simulink model "lss"  (R2022b)
settings: Solver=FixedStepAuto  StartTime=0.0  StopTime=Inf  FixedStep=0.001  RelTol=1e-3  EnableMultiTasking=on
InitFcn:
  | clear mex
model workspace (MAT data in the model file):
  worldsim_instance : object (value not decoded)
values from neighbouring files (symbols this model uses):
  ADAS_Control_Mode = 1    [LSS_parameters.m]    (also in lss_ini_param.sldd = 1.0)
  butter_a = 1.0 -1.9911142922016536 0.99115359586893548    [lss_ini_param.sldd]
  butter_a_lka_out = 1.0 -1.5610180758007179 0.641351538057563    [lss_ini_param.sldd]
  butter_b = 9.825916820482009E-6 1.9651833640964018E-5 9.825916820482009E-6    [lss_ini_param.sldd]
  butter_b_lka_out = 0.020083365564211246 0.040166731128422492 0.020083365564211246    [lss_ini_param.sldd]
  index_variant_approaching_speed = 3.0    [lss_ini_param.sldd]
  initCond = vi_worldsim_load_scenario(worldsim_process,scenario_path,'lss_online')    [launcher.m]
  LDW_Activity_Flag = 1    [LSS_parameters.m]    (also in lss_ini_param.sldd = 1.0)
  LDW_Freq_Hz = Sensor_Freq_worldsim    [LSS_parameters.m]    (also in lss_ini_param.sldd = 50.0)
  LDW_LaneGap_dydt_Warning = 50    [LSS_parameters.m]    (also in lss_ini_param.sldd = 50.0)
  LDW_LaneGap_Warning = [0.5 0.25]    [LSS_parameters.m]    (also in lss_ini_param.sldd = 0.5 0.25)
  LDW_Min_Speed = 60    [LSS_parameters.m]    (also in lss_ini_param.sldd = 60.0)
  LDW_Steer_Vibration_Amplitude = 5    [LSS_parameters.m]    (also in lss_ini_param.sldd = 5.0)
  LDW_Steer_Vibration_Freq = 25    [LSS_parameters.m]    (also in lss_ini_param.sldd = 25.0)
  LKA_Activity_Flag = 1    [LSS_parameters.m]    (also in lss_ini_param.sldd = 1.0)
  LKA_D = [0.2 0.3]    [LSS_parameters.m]    (also in lss_ini_param.sldd = 0.2 0.3)
  LKA_Dyn_Rate_Limiter_Gain = 0.1    [LSS_parameters.m]    (also in lss_ini_param.sldd)
  LKA_Dyn_Rate_Limiter_Power = 10    [LSS_parameters.m]    (also in lss_ini_param.sldd = 10.0)
  LKA_Error_dydt_Off = 1    [LSS_parameters.m]    (also in lss_ini_param.sldd = 1.0)
  LKA_Error_Max = 3    [LSS_parameters.m]    (also in lss_ini_param.sldd = 3.0)
  LKA_Error_Off = 0.5    [LSS_parameters.m]    (also in lss_ini_param.sldd)
  LKA_Freq_Hz = Sensor_Freq_worldsim    [LSS_parameters.m]    (also in lss_ini_param.sldd = 50.0)
  LKA_I = [0.025 0.05]    [LSS_parameters.m]    (also in lss_ini_param.sldd = 0.025 0.05)
  LKA_Lane_Gap_Activate = [0.25 0.125]    [LSS_parameters.m]    (also in lss_ini_param.sldd = -0.05 0.125)
  LKA_Lane_Gap_dydt_Activate = 50    [LSS_parameters.m]    (also in lss_ini_param.sldd = 50.0)
  LKA_Min_Speed = 60    [LSS_parameters.m]    (also in lss_ini_param.mat = 50; lss_ini_param.sldd = 50.0)
  LKA_On_Display_Freq = 5    [LSS_parameters.m]    (also in lss_ini_param.sldd = 5.0)
  LKA_P = [0.1 0.2]    [LSS_parameters.m]    (also in lss_ini_param.sldd = 0.1 0.2)
  LKA_Steer_Rate_Max_radps = 1    [LSS_parameters.m]    (also in lss_ini_param.sldd = 1.0)
  radar_source = 2    [LSS_parameters.m]    (also in lss_ini_param.sldd = 2.0)
  Sensor_Freq_worldsim = 50    [launcher.m]    (also in lss_ini_param.sldd = 50.0)
  simulation_crt = '../VI-CarRealTime_model/SedanCar_WorldSim_Offline_send_svm.xml'    [launcher.m]
  stop_number_collisions = 5    [launcher.m]
  stop_speed = 0.001    [launcher.m]
  stop_time = 20    [launcher.m]
  target_speed = 72    [LSS_parameters.m]    (also in launcher.m = initCond.initialVelocity * 3.6)
  variant_approaching_speed = v_lat    [launcher.m]    (also in lss_ini_param.sldd = 0.2 0.3 0.4 0.5 0.6)
  vehicle_width = 1.86    [LSS_parameters.m]    (also in lss_ini_param.sldd = 2.05)
undefined symbols (not defined in the file or in its folder): Driver_Demands, light_brake_center, light_brake_left, light_brake_right, steer_assist, vicrt_initcallback, vicrt_initmexcallback, vicrt_simulationmanager
libraries: simulink x39, simwbSfunlib x15, viworldsim_lib x5
(part 6 of 6)

== system lss/VI-CarRealTime/Input_Bus/Inputs/Main_Spring/force ==
  BCforce : BusCreator  Inputs=4
  L1_def_val : Constant  Value=0
  L2_def_val : Constant  Value=0
  R1_def_val : Constant  Value=0
  R2_def_val : Constant  Value=0
  force : Outport
  wires:
  BCforce/1 -> force/1  "force"
  L1_def_val/1 -> BCforce/1  "L1"
  L2_def_val/1 -> BCforce/2  "L2"
  R1_def_val/1 -> BCforce/3  "R1"
  R2_def_val/1 -> BCforce/4  "R2"

== system lss/VI-CarRealTime/Input_Bus/Inputs/Mono_Element/Bumpstop_Damper ==
  BCBumpstop_Damper : BusCreator  Inputs=2
  front_def_val : Constant  Value=0
  rear_def_val : Constant  Value=0
  Bumpstop_Damper : Outport
  wires:
  BCBumpstop_Damper/1 -> Bumpstop_Damper/1  "Bumpstop_Damper"
  front_def_val/1 -> BCBumpstop_Damper/1  "front"
  rear_def_val/1 -> BCBumpstop_Damper/2  "rear"

== system lss/VI-CarRealTime/Input_Bus/Inputs/Mono_Element/Bumpstop_Damper_activity_flag ==
  BCBumpstop_Damper_activity_flag : BusCreator  Inputs=2
  front_def_val : Constant
  rear_def_val : Constant
  Bumpstop_Damper_activity_flag : Outport
  wires:
  BCBumpstop_Damper_activity_flag/1 -> Bumpstop_Damper_activity_flag/1  "Bumpstop_Damper_activity_flag"
  front_def_val/1 -> BCBumpstop_Damper_activity_flag/1  "front"
  rear_def_val/1 -> BCBumpstop_Damper_activity_flag/2  "rear"

== system lss/VI-CarRealTime/Input_Bus/Inputs/Mono_Element/Bumpstop_Spring ==
  BCBumpstop_Spring : BusCreator  Inputs=2
  front_def_val : Constant  Value=0
  rear_def_val : Constant  Value=0
  Bumpstop_Spring : Outport
  wires:
  BCBumpstop_Spring/1 -> Bumpstop_Spring/1  "Bumpstop_Spring"
  front_def_val/1 -> BCBumpstop_Spring/1  "front"
  rear_def_val/1 -> BCBumpstop_Spring/2  "rear"

== system lss/VI-CarRealTime/Input_Bus/Inputs/Mono_Element/Bumpstop_Spring_activity_flag ==
  BCBumpstop_Spring_activity_flag : BusCreator  Inputs=2
  front_def_val : Constant
  rear_def_val : Constant
  Bumpstop_Spring_activity_flag : Outport
  wires:
  BCBumpstop_Spring_activity_flag/1 -> Bumpstop_Spring_activity_flag/1  "Bumpstop_Spring_activity_flag"
  front_def_val/1 -> BCBumpstop_Spring_activity_flag/1  "front"
  rear_def_val/1 -> BCBumpstop_Spring_activity_flag/2  "rear"

== system lss/VI-CarRealTime/Input_Bus/Inputs/Mono_Element/Damper ==
  BCDamper : BusCreator  Inputs=2
  front_def_val : Constant  Value=0
  rear_def_val : Constant  Value=0
  Damper : Outport
  wires:
  BCDamper/1 -> Damper/1  "Damper"
  front_def_val/1 -> BCDamper/1  "front"
  rear_def_val/1 -> BCDamper/2  "rear"

== system lss/VI-CarRealTime/Input_Bus/Inputs/Mono_Element/Damper_activity_flag ==
  BCDamper_activity_flag : BusCreator  Inputs=2
  front_def_val : Constant
  rear_def_val : Constant
  Damper_activity_flag : Outport
  wires:
  BCDamper_activity_flag/1 -> Damper_activity_flag/1  "Damper_activity_flag"
  front_def_val/1 -> BCDamper_activity_flag/1  "front"
  rear_def_val/1 -> BCDamper_activity_flag/2  "rear"

== system lss/VI-CarRealTime/Input_Bus/Inputs/Mono_Element/Inerter ==
  BCInerter : BusCreator  Inputs=2
  front_def_val : Constant  Value=0
  rear_def_val : Constant  Value=0
  Inerter : Outport
  wires:
  BCInerter/1 -> Inerter/1  "Inerter"
  front_def_val/1 -> BCInerter/1  "front"
  rear_def_val/1 -> BCInerter/2  "rear"

== system lss/VI-CarRealTime/Input_Bus/Inputs/Mono_Element/Inerter_activity_flag ==
  BCInerter_activity_flag : BusCreator  Inputs=2
  front_def_val : Constant
  rear_def_val : Constant
  Inerter_activity_flag : Outport
  wires:
  BCInerter_activity_flag/1 -> Inerter_activity_flag/1  "Inerter_activity_flag"
  front_def_val/1 -> BCInerter_activity_flag/1  "front"
  rear_def_val/1 -> BCInerter_activity_flag/2  "rear"

== system lss/VI-CarRealTime/Input_Bus/Inputs/Mono_Element/Reboundstop_Damper ==
  BCReboundstop_Damper : BusCreator  Inputs=2
  front_def_val : Constant  Value=0
  rear_def_val : Constant  Value=0
  Reboundstop_Damper : Outport
  wires:
  BCReboundstop_Damper/1 -> Reboundstop_Damper/1  "Reboundstop_Damper"
  front_def_val/1 -> BCReboundstop_Damper/1  "front"
  rear_def_val/1 -> BCReboundstop_Damper/2  "rear"

== system lss/VI-CarRealTime/Input_Bus/Inputs/Mono_Element/Reboundstop_Damper_activity_flag ==
  BCReboundstop_Damper_activity_flag : BusCreator  Inputs=2
  front_def_val : Constant
  rear_def_val : Constant
  Reboundstop_Damper_activity_flag : Outport
  wires:
  BCReboundstop_Damper_activity_flag/1 -> Reboundstop_Damper_activity_flag/1  "Reboundstop_Damper_activity_flag"
  front_def_val/1 -> BCReboundstop_Damper_activity_flag/1  "front"
  rear_def_val/1 -> BCReboundstop_Damper_activity_flag/2  "rear"

== system lss/VI-CarRealTime/Input_Bus/Inputs/Mono_Element/Reboundstop_Spring ==
  BCReboundstop_Spring : BusCreator  Inputs=2
  front_def_val : Constant  Value=0
  rear_def_val : Constant  Value=0
  Reboundstop_Spring : Outport
  wires:
  BCReboundstop_Spring/1 -> Reboundstop_Spring/1  "Reboundstop_Spring"
  front_def_val/1 -> BCReboundstop_Spring/1  "front"
  rear_def_val/1 -> BCReboundstop_Spring/2  "rear"

== system lss/VI-CarRealTime/Input_Bus/Inputs/Mono_Element/Reboundstop_Spring_activity_flag ==
  BCReboundstop_Spring_activity_flag : BusCreator  Inputs=2
  front_def_val : Constant
  rear_def_val : Constant
  Reboundstop_Spring_activity_flag : Outport
  wires:
  BCReboundstop_Spring_activity_flag/1 -> Reboundstop_Spring_activity_flag/1  "Reboundstop_Spring_activity_flag"
  front_def_val/1 -> BCReboundstop_Spring_activity_flag/1  "front"
  rear_def_val/1 -> BCReboundstop_Spring_activity_flag/2  "rear"

== system lss/VI-CarRealTime/Input_Bus/Inputs/Mono_Element/Roll_Damper ==
  BCRoll_Damper : BusCreator  Inputs=2
  front_def_val : Constant  Value=0
  rear_def_val : Constant  Value=0
  Roll_Damper : Outport
  wires:
  BCRoll_Damper/1 -> Roll_Damper/1  "Roll_Damper"
  front_def_val/1 -> BCRoll_Damper/1  "front"
  rear_def_val/1 -> BCRoll_Damper/2  "rear"

== system lss/VI-CarRealTime/Input_Bus/Inputs/Mono_Element/Roll_Damper_activity_flag ==
  BCRoll_Damper_activity_flag : BusCreator  Inputs=2
  front_def_val : Constant
  rear_def_val : Constant
  Roll_Damper_activity_flag : Outport
  wires:
  BCRoll_Damper_activity_flag/1 -> Roll_Damper_activity_flag/1  "Roll_Damper_activity_flag"
  front_def_val/1 -> BCRoll_Damper_activity_flag/1  "front"
  rear_def_val/1 -> BCRoll_Damper_activity_flag/2  "rear"

== system lss/VI-CarRealTime/Input_Bus/Inputs/Mono_Element/Spring ==
  BCSpring : BusCreator  Inputs=2
  front_def_val : Constant  Value=0
  rear_def_val : Constant  Value=0
  Spring : Outport
  wires:
  BCSpring/1 -> Spring/1  "Spring"
  front_def_val/1 -> BCSpring/1  "front"
  rear_def_val/1 -> BCSpring/2  "rear"

== system lss/VI-CarRealTime/Input_Bus/Inputs/Mono_Element/Spring_activity_flag ==
  BCSpring_activity_flag : BusCreator  Inputs=2
  front_def_val : Constant
  rear_def_val : Constant
  Spring_activity_flag : Outport
  wires:
  BCSpring_activity_flag/1 -> Spring_activity_flag/1  "Spring_activity_flag"
  front_def_val/1 -> BCSpring_activity_flag/1  "front"
  rear_def_val/1 -> BCSpring_activity_flag/2  "rear"

== system lss/VI-CarRealTime/Input_Bus/Inputs/Rear_Steering_Actuator_disp/str_swa ==
  BCstr_swa : BusCreator  Inputs=2
  left_def_val : Constant  Value=0
  right_def_val : Constant  Value=0
  str_swa : Outport
  wires:
  BCstr_swa/1 -> str_swa/1  "str_swa"
  left_def_val/1 -> BCstr_swa/1  "left"
  right_def_val/1 -> BCstr_swa/2  "right"

== system lss/VI-CarRealTime/Input_Bus/Inputs/Steering/steer_at_spindle ==
  BCsteer_at_spindle : BusCreator  Inputs=4
  L1_def_val : Constant  Value=0
  L2_def_val : Constant  Value=0
  R1_def_val : Constant  Value=0
  R2_def_val : Constant  Value=0
  steer_at_spindle : Outport
  wires:
  BCsteer_at_spindle/1 -> steer_at_spindle/1  "steer_at_spindle"
  L1_def_val/1 -> BCsteer_at_spindle/1  "L1"
  L2_def_val/1 -> BCsteer_at_spindle/2  "L2"
  R1_def_val/1 -> BCsteer_at_spindle/3  "R1"
  R2_def_val/1 -> BCsteer_at_spindle/4  "R2"

== system lss/VI-CarRealTime/Input_Bus/Inputs/Subsystem_Activation/Internal_Brake_System_Activity ==
  BCInternal_Brake_System_Activity : BusCreator  Inputs=4
  L1_def_val : Constant
  L2_def_val : Constant
  R1_def_val : Constant
  R2_def_val : Constant
  Internal_Brake_System_Activity : Outport
  wires:
  BCInternal_Brake_System_Activity/1 -> Internal_Brake_System_Activity/1  "Internal_Brake_System_Activity"
  L1_def_val/1 -> BCInternal_Brake_System_Activity/1  "L1"
  L2_def_val/1 -> BCInternal_Brake_System_Activity/2  "L2"
  R1_def_val/1 -> BCInternal_Brake_System_Activity/3  "R1"
  R2_def_val/1 -> BCInternal_Brake_System_Activity/4  "R2"

== system lss/VI-CarRealTime/Input_Bus/Inputs/Subsystem_Activation/Tire_Force_x ==
  BCTire_Force_x : BusCreator  Inputs=4
  L1_def_val : Constant
  L2_def_val : Constant
  R1_def_val : Constant
  R2_def_val : Constant
  Tire_Force_x : Outport
  wires:
  BCTire_Force_x/1 -> Tire_Force_x/1  "Tire_Force_x"
  L1_def_val/1 -> BCTire_Force_x/1  "L1"
  L2_def_val/1 -> BCTire_Force_x/2  "L2"
  R1_def_val/1 -> BCTire_Force_x/3  "R1"
  R2_def_val/1 -> BCTire_Force_x/4  "R2"

== system lss/VI-CarRealTime/Input_Bus/Inputs/Subsystem_Activation/Tire_Force_y ==
  BCTire_Force_y : BusCreator  Inputs=4
  L1_def_val : Constant
  L2_def_val : Constant
  R1_def_val : Constant
  R2_def_val : Constant
  Tire_Force_y : Outport
  wires:
  BCTire_Force_y/1 -> Tire_Force_y/1  "Tire_Force_y"
  L1_def_val/1 -> BCTire_Force_y/1  "L1"
  L2_def_val/1 -> BCTire_Force_y/2  "L2"
  R1_def_val/1 -> BCTire_Force_y/3  "R1"
  R2_def_val/1 -> BCTire_Force_y/4  "R2"

== system lss/VI-CarRealTime/Input_Bus/Inputs/Subsystem_Activation/Tire_Force_z ==
  BCTire_Force_z : BusCreator  Inputs=4
  L1_def_val : Constant
  L2_def_val : Constant
  R1_def_val : Constant
  R2_def_val : Constant
  Tire_Force_z : Outport
  wires:
  BCTire_Force_z/1 -> Tire_Force_z/1  "Tire_Force_z"
  L1_def_val/1 -> BCTire_Force_z/1  "L1"
  L2_def_val/1 -> BCTire_Force_z/2  "L2"
  R1_def_val/1 -> BCTire_Force_z/3  "R1"
  R2_def_val/1 -> BCTire_Force_z/4  "R2"

== system lss/VI-CarRealTime/Input_Bus/Inputs/Subsystem_Activation/Tire_Moment_x ==
  BCTire_Moment_x : BusCreator  Inputs=4
  L1_def_val : Constant
  L2_def_val : Constant
  R1_def_val : Constant
  R2_def_val : Constant
  Tire_Moment_x : Outport
  wires:
  BCTire_Moment_x/1 -> Tire_Moment_x/1  "Tire_Moment_x"
  L1_def_val/1 -> BCTire_Moment_x/1  "L1"
  L2_def_val/1 -> BCTire_Moment_x/2  "L2"
  R1_def_val/1 -> BCTire_Moment_x/3  "R1"
  R2_def_val/1 -> BCTire_Moment_x/4  "R2"

== system lss/VI-CarRealTime/Input_Bus/Inputs/Subsystem_Activation/Tire_Moment_y ==
  BCTire_Moment_y : BusCreator  Inputs=4
  L1_def_val : Constant
  L2_def_val : Constant
  R1_def_val : Constant
  R2_def_val : Constant
  Tire_Moment_y : Outport
  wires:
  BCTire_Moment_y/1 -> Tire_Moment_y/1  "Tire_Moment_y"
  L1_def_val/1 -> BCTire_Moment_y/1  "L1"
  L2_def_val/1 -> BCTire_Moment_y/2  "L2"
  R1_def_val/1 -> BCTire_Moment_y/3  "R1"
  R2_def_val/1 -> BCTire_Moment_y/4  "R2"

== system lss/VI-CarRealTime/Input_Bus/Inputs/Subsystem_Activation/Tire_Moment_z ==
  BCTire_Moment_z : BusCreator  Inputs=4
  L1_def_val : Constant
  L2_def_val : Constant
  R1_def_val : Constant
  R2_def_val : Constant
  Tire_Moment_z : Outport
  wires:
  BCTire_Moment_z/1 -> Tire_Moment_z/1  "Tire_Moment_z"
  L1_def_val/1 -> BCTire_Moment_z/1  "L1"
  L2_def_val/1 -> BCTire_Moment_z/2  "L2"
  R1_def_val/1 -> BCTire_Moment_z/3  "R1"
  R2_def_val/1 -> BCTire_Moment_z/4  "R2"

== system lss/VI-CarRealTime/Input_Bus/Inputs/Third_Element/Damper_activity_flag ==
  BCDamper_activity_flag : BusCreator  Inputs=2
  front_def_val : Constant
  rear_def_val : Constant
  Damper_activity_flag : Outport
  wires:
  BCDamper_activity_flag/1 -> Damper_activity_flag/1  "Damper_activity_flag"
  front_def_val/1 -> BCDamper_activity_flag/1  "front"
  rear_def_val/1 -> BCDamper_activity_flag/2  "rear"

== system lss/VI-CarRealTime/Input_Bus/Inputs/Third_Element/Damper_force ==
  BCDamper_force : BusCreator  Inputs=2
  front_def_val : Constant  Value=0
  rear_def_val : Constant  Value=0
  Damper_force : Outport
  wires:
  BCDamper_force/1 -> Damper_force/1  "Damper_force"
  front_def_val/1 -> BCDamper_force/1  "front"
  rear_def_val/1 -> BCDamper_force/2  "rear"

== system lss/VI-CarRealTime/Input_Bus/Inputs/Third_Element/Spring ==
  BCSpring : BusCreator  Inputs=2
  front_def_val : Constant  Value=0
  rear_def_val : Constant  Value=0
  Spring : Outport
  wires:
  BCSpring/1 -> Spring/1  "Spring"
  front_def_val/1 -> BCSpring/1  "front"
  rear_def_val/1 -> BCSpring/2  "rear"

== system lss/VI-CarRealTime/Input_Bus/Inputs/Third_Element/Spring_activity_flag ==
  BCSpring_activity_flag : BusCreator  Inputs=2
  front_def_val : Constant
  rear_def_val : Constant
  Spring_activity_flag : Outport
  wires:
  BCSpring_activity_flag/1 -> Spring_activity_flag/1  "Spring_activity_flag"
  front_def_val/1 -> BCSpring_activity_flag/1  "front"
  rear_def_val/1 -> BCSpring_activity_flag/2  "rear"

== system lss/VI-CarRealTime/Input_Bus/Inputs/Tire_Force/Fx ==
  BCFx : BusCreator  Inputs=4
  L1_def_val : Constant  Value=0
  L2_def_val : Constant  Value=0
  R1_def_val : Constant  Value=0
  R2_def_val : Constant  Value=0
  Fx : Outport
  wires:
  BCFx/1 -> Fx/1  "Fx"
  L1_def_val/1 -> BCFx/1  "L1"
  L2_def_val/1 -> BCFx/2  "L2"
  R1_def_val/1 -> BCFx/3  "R1"
  R2_def_val/1 -> BCFx/4  "R2"

== system lss/VI-CarRealTime/Input_Bus/Inputs/Tire_Force/Fy ==
  BCFy : BusCreator  Inputs=4
  L1_def_val : Constant  Value=0
  L2_def_val : Constant  Value=0
  R1_def_val : Constant  Value=0
  R2_def_val : Constant  Value=0
  Fy : Outport
  wires:
  BCFy/1 -> Fy/1  "Fy"
  L1_def_val/1 -> BCFy/1  "L1"
  L2_def_val/1 -> BCFy/2  "L2"
  R1_def_val/1 -> BCFy/3  "R1"
  R2_def_val/1 -> BCFy/4  "R2"

== system lss/VI-CarRealTime/Input_Bus/Inputs/Tire_Force/Fz ==
  BCFz : BusCreator  Inputs=4
  L1_def_val : Constant  Value=0
  L2_def_val : Constant  Value=0
  R1_def_val : Constant  Value=0
  R2_def_val : Constant  Value=0
  Fz : Outport
  wires:
  BCFz/1 -> Fz/1  "Fz"
  L1_def_val/1 -> BCFz/1  "L1"
  L2_def_val/1 -> BCFz/2  "L2"
  R1_def_val/1 -> BCFz/3  "R1"
  R2_def_val/1 -> BCFz/4  "R2"

== system lss/VI-CarRealTime/Input_Bus/Inputs/Tire_Moment/Mx ==
  BCMx : BusCreator  Inputs=4
  L1_def_val : Constant  Value=0
  L2_def_val : Constant  Value=0
  R1_def_val : Constant  Value=0
  R2_def_val : Constant  Value=0
  Mx : Outport
  wires:
  BCMx/1 -> Mx/1  "Mx"
  L1_def_val/1 -> BCMx/1  "L1"
  L2_def_val/1 -> BCMx/2  "L2"
  R1_def_val/1 -> BCMx/3  "R1"
  R2_def_val/1 -> BCMx/4  "R2"

== system lss/VI-CarRealTime/Input_Bus/Inputs/Tire_Moment/My ==
  BCMy : BusCreator  Inputs=4
  L1_def_val : Constant  Value=0
  L2_def_val : Constant  Value=0
  R1_def_val : Constant  Value=0
  R2_def_val : Constant  Value=0
  My : Outport
  wires:
  BCMy/1 -> My/1  "My"
  L1_def_val/1 -> BCMy/1  "L1"
  L2_def_val/1 -> BCMy/2  "L2"
  R1_def_val/1 -> BCMy/3  "R1"
  R2_def_val/1 -> BCMy/4  "R2"

== system lss/VI-CarRealTime/Input_Bus/Inputs/Tire_Moment/Mz ==
  BCMz : BusCreator  Inputs=4
  L1_def_val : Constant  Value=0
  L2_def_val : Constant  Value=0
  R1_def_val : Constant  Value=0
  R2_def_val : Constant  Value=0
  Mz : Outport
  wires:
  BCMz/1 -> Mz/1  "Mz"
  L1_def_val/1 -> BCMz/1  "L1"
  L2_def_val/1 -> BCMz/2  "L2"
  R1_def_val/1 -> BCMz/3  "R1"
  R2_def_val/1 -> BCMz/4  "R2"

== system lss/VI-CarRealTime/Input_Bus/Inputs/Wheel_driving/moment ==
  BCmoment : BusCreator  Inputs=4
  L1_def_val : Constant  Value=0
  L2_def_val : Constant  Value=0
  R1_def_val : Constant  Value=0
  R2_def_val : Constant  Value=0
  moment : Outport
  wires:
  BCmoment/1 -> moment/1  "moment"
  L1_def_val/1 -> BCmoment/1  "L1"
  L2_def_val/1 -> BCmoment/2  "L2"
  R1_def_val/1 -> BCmoment/3  "R1"
  R2_def_val/1 -> BCmoment/4  "R2"

== matlab function lss/OUTPUT/WorldSim_Sensor_Outputs/manipulation_of_objects1 ==
  data: complete_obstacles_matrix input; filtered_matrix output; detected_objects input
function filtered_matrix = fcn(complete_obstacles_matrix, detected_objects)

% computations

filtered_matrix = complete_obstacles_matrix;

filtered_matrix(:,((detected_objects+1):size(filtered_matrix,2))) = 0;

== matlab function lss/LKA/MATLAB Function ==
  data: u input; y output
function y = fcn(u)

if u == 0
    y=1e-6;
else
    y=u;
end

end

== matlab function lss/OUTPUT/WorldSim_Sensor_Outputs/MATLAB Function ==
  data: lane_coefficiants input; left_lane_distance output; right_lane_distance output
function [left_lane_distance, right_lane_distance] = fcn(lane_coefficiants)

left_lane_distance = lane_coefficiants(1,1);
right_lane_distance = lane_coefficiants(2,1);

== matlab function lss/OUTPUT/WorldSim_Sensor_Outputs/manipulation_of_objects ==
  data: complete_obstacles_matrix input; filtered_matrix output; detected_objects input
function filtered_matrix = fcn(complete_obstacles_matrix, detected_objects)

% computations

filtered_matrix = complete_obstacles_matrix;

filtered_matrix(:,((detected_objects+1):size(filtered_matrix,2))) = 0;

== matlab function lss/OUTPUT/WorldSim_Sensor_Outputs/Subsystem/multiagent radar SimpleRadar_... are single double representing id, yaw, range, power_db, range_rate, yaw_rate, status/MATLAB Function1 ==
  data: u input; id output; yaw output; range output; power_db output; range_rate output; yaw_rate output; status output
function [id, yaw, range, power_db, range_rate, yaw_rate,status] = fcn(u)

id = u(:,1);
yaw = u(:,2);
range = u(:,3);
power_db = u(:,4);
range_rate = u(:,5);
yaw_rate = u(:,6);
status = u(:,7);

== matlab function lss/OUTPUT/WorldSim_Sensor_Outputs/Subsystem/obstacle detection /MATLAB Function2 ==
  data: u input; tag output; center_x output; center_y output; center_z output; center_rotation_x output; center_rotation_y output; center_rotation_z output; size_x output; size_y output; size_z output
function [tag, center_x, center_y, center_z, center_rotation_x, center_rotation_y, center_rotation_z, size_x, size_y, size_z] = fcn(u)

% this is the id tag that is assigned by ws at every scenario load
tag = (u(1,:))';
center_x = (u(2,:))';
center_y = (u(3,:))';
center_z = (u(4,:))';
center_rotation_x = (u(5,:))';
center_rotation_y = (u(6,:))';
center_rotation_z = (u(7,:))';
size_x = (u(8,:))';
size_y = (u(9,:))';
size_z = (u(10,:))';

%% identification of nearest box

% [index,index2]=min(u(:,3));
% 
% id = u(index,1);
% type = u(index,2);
% center_x = u(index,3);
% center_y = u(index,4);
% center_z = u(index,5);
% width = u(index,6);
% height = u(index,7);

== matlab function lss/OUTPUT/WorldSim_Sensor_Outputs/Subsystem/obstacle detection /MATLAB Function ==
  data: x input; distanceToCollision output; y input; yaw output
function [distanceToCollision, yaw] = fcn(x, y)

x(x==0)=121;
y(y==0)=121;

yaw = atan(y./x);
distanceToCollision=x./cos(yaw);
distanceToCollision(x==121)=121;

== matlab function lss/OUTPUT/WorldSim_Sensor_Outputs/Subsystem/bsd setection from ostacle recognition/MATLAB Function3 ==
  data: u input; semitrack input; left output; right output
function [left, right] = fcn(u, semitrack)
left=0;
right=0;

% [x,index] = min(nonzeros(u(:,3)));
x = (u(2,:))';
y = (u(3,:))';
% yaw = atan(y./x);
% distanceToCollision=x./cos(yaw);
index_left=find((y < -semitrack).*(y > -5),1);
index_right=find((y > semitrack).*(y < 5),1);
% .*(y > -3).*(x < 25)
if (~isempty(index_left))
    left = 1;
end
if (~isempty(index_right))
    right=1;
end
